simulink model "35-Bus_Network_Electricity_Transmission_Model"  (R2023b)
settings: Solver=VariableStepAuto  StartTime=0.0  StopTime=10  RelTol=1e-3
undefined symbols (not defined in the file): D1, D11, Delta
libraries: spsSeriesRLCBranchLib x47, spsLoadFlowBusLib x35, spsThreePhaseSeriesRLCLoadLib x27, spsDistributedParametersLineLib x22, spsGenericPowerSystemStabilizerLib x20, spsThreePhaseTransformerTwoWindingsLib x19, spsThreePhaseVIMeasurementLib x13, spsSynchronousMachinepuStandardLib x10, spsExcitationSystemLib x10, spsHydraulicTurbineandGovernorLib x10, spsThreePhaseParallelRLCLoadLib x4, spsGroundLib x3
(part 2 of 7)

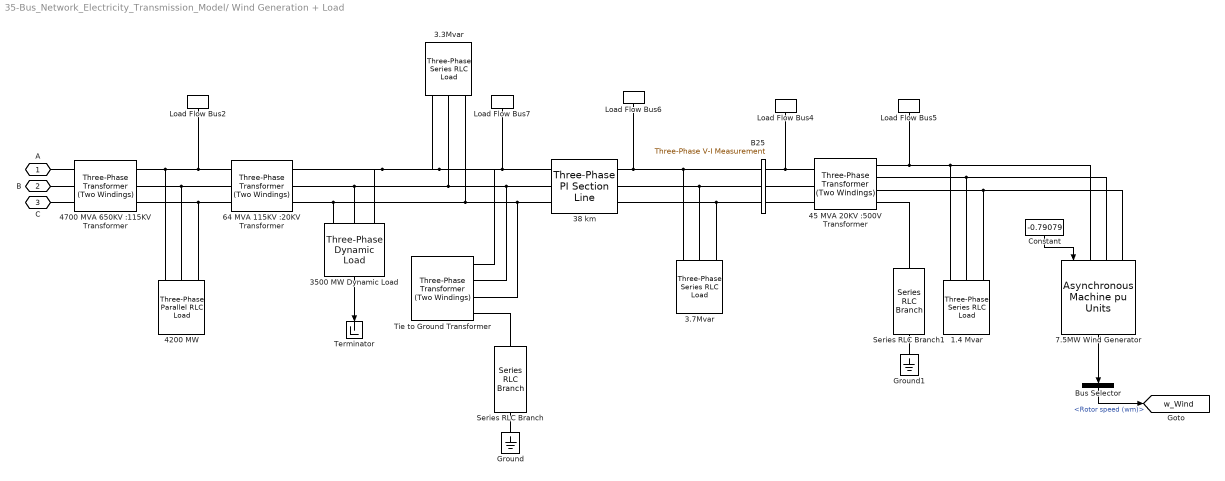
== system 35-Bus_Network_Electricity_Transmission_Model/ Wind Generation + Load ==
  " 64 MVA 115KV :20KV Transformer " : spsThreePhaseTransformerTwoWindingsLib/Three-Phase Transformer (Two Windings)  Winding1Connection=Yg  Winding2Connection=Delta (D1)  CoreType=Three single-phase transformers  SetSaturation=off  Hysteresis=off  DataFile='hysteresis'  SetInitialFlux=off  Measurements=None  UNITS=pu  NominalPower=[ 64e6 , 60 ]  Winding1=[ 115e3 , 0.002 , 0.08 ]  Winding2=[ 20e3 , 0.002 , 0.08 ]  Rm=500  Lm=500  L0=0.5  Saturation=[ 0,0 ; 0.0024,1.2 ; 1.0,1.52 ]  InitialFluxes=[ 0.8 , -0.8 , 0.7 ]  BreakLoop=off  DiscreteSolver=Trapezoidal iterative  DataType=off  TransfoNumber=1
  " Tie to Ground Transformer " : spsThreePhaseTransformerTwoWindingsLib/Three-Phase Transformer (Two Windings)  Winding1Connection=Yn  Winding2Connection=Delta (D11)  CoreType=Three single-phase transformers  SetSaturation=off  Hysteresis=off  DataFile='hysteresis'  SetInitialFlux=off  Measurements=None  UNITS=pu  NominalPower=[ 5600e6 , 60 ]  Winding1=[ 13.8e3 , 0.002 , 0.08 ]  Winding2=[ 735e3 , 0.002 , 0.08 ]  Rm=500  Lm=500  L0=0.5  Saturation=[ 0,0 ; 0.0024,1.2 ; 1.0,1.52 ]  InitialFluxes=[ 0.8 , -0.8 , 0.7 ]  BreakLoop=off  DiscreteSolver=Trapezoidal iterative  DataType=off  TransfoNumber=1
  1.4 Mvar : spsThreePhaseSeriesRLCLoadLib/Three-Phase Series RLC Load  LConnTagsString=A|B|C  Configuration=Y (grounded)  NominalVoltage=1000  Vabc=[1e3 1e3 1e3]  Vabcp=[1e3 1e3 1e3]  NominalFrequency=60  UnbalancedPower=off  ActivePower=0  InductivePower=0  CapacitivePower=1.4e6  Pabc=[10e3 9e3 11e3]  QLabc=[100 90 110]  QCabc=[100 90 110]  Pabcp=[10e3 9e3 11e3]  QLabcp=[100 90 110]  QCabcp=[100 90 110]  Measurements=None  LoadType=constant Z
  3.3Mvar : spsThreePhaseSeriesRLCLoadLib/Three-Phase Series RLC Load  LConnTagsString=A|B|C  Configuration=Y (grounded)  NominalVoltage=1000  Vabc=[1e3 1e3 1e3]  Vabcp=[1e3 1e3 1e3]  NominalFrequency=60  UnbalancedPower=off  ActivePower=0  InductivePower=0  CapacitivePower=3.3e6  Pabc=[10e3 9e3 11e3]  QLabc=[100 90 110]  QCabc=[100 90 110]  Pabcp=[10e3 9e3 11e3]  QLabcp=[100 90 110]  QCabcp=[100 90 110]  Measurements=None  LoadType=constant Z
  3.7Mvar : spsThreePhaseSeriesRLCLoadLib/Three-Phase Series RLC Load  LConnTagsString=A|B|C  Configuration=Y (grounded)  NominalVoltage=1000  Vabc=[1e3 1e3 1e3]  Vabcp=[1e3 1e3 1e3]  NominalFrequency=60  UnbalancedPower=off  ActivePower=0  InductivePower=0  CapacitivePower=3.7e6  Pabc=[10e3 9e3 11e3]  QLabc=[100 90 110]  QCabc=[100 90 110]  Pabcp=[10e3 9e3 11e3]  QLabcp=[100 90 110]  QCabcp=[100 90 110]  Measurements=None  LoadType=constant Z
  3500 MW Dynamic Load : spsThreePhaseDynamicLoadLib/Three-Phase Dynamic Load  NominalVoltage=[ 500e3 60 ]  ActiveReactivePowers=[3500e6 0]  PositiveSequence=[0.994 -11.8]  ExternalControl=off  NpNq=[1.3 2]  TimeConstants="[0  0  0  0]"  MinimumVoltage=0.7  Tfilter=1e-4  LoadFlowParameters=[4,0,0,0,0]
      settings: LibrarySourceBlock=|
      | sps_lib/Passives/Three-Phase
      | Dynamic Load
  38 km : spsThreePhasePISectionLineLib/Three-Phase PI Section Line  LConnTagsString=a|b|c  RConnTagsString=A|B|C  Length=38  Frequency=60  Resistances=[ 0.01273 0.3864]/6  Inductances="[ 0.9337e-3  4.1264e-3]/6"  Capacitances=[12.74e-9 7.751e-9]*6
  4200 MW : spsThreePhaseParallelRLCLoadLib/Three-Phase Parallel RLC Load  LConnTagsString=A|B|C  Configuration=Y (grounded)  NominalVoltage=1000  Vabc=[1e3 1e3 1e3]  Vabcp=[1e3 1e3 1e3]  NominalFrequency=60  UnbalancedPower=off  ActivePower=4200e6  InductivePower=0  CapacitivePower=0  Pabc=[10e3 9e3 11e3]  QLabc=[100 90 110]  QCabc=[100 90 110]  Pabcp=[10e3 9e3 11e3]  QLabcp=[100 90 110]  QCabcp=[100 90 110]  Measurements=None  LoadType=constant Z
  "45 MVA 20KV :500V Transformer " : spsThreePhaseTransformerTwoWindingsLib/Three-Phase Transformer (Two Windings)  Winding1Connection=Yg  Winding2Connection=Yn  CoreType=Three single-phase transformers  SetSaturation=off  Hysteresis=off  DataFile='hysteresis'  SetInitialFlux=off  Measurements=None  UNITS=pu  NominalPower=[ 12e6 , 60 ]  Winding1=[ 20e3 , 0.002 , 0.08 ]  Winding2=[ 500 , 0.002 , 0.08 ]  Rm=500  Lm=500  L0=0.5  Saturation=[ 0,0 ; 0.0024,1.2 ; 1.0,1.52 ]  InitialFluxes=[ 0.8 , -0.8 , 0.7 ]  BreakLoop=off  DiscreteSolver=Trapezoidal iterative  DataType=off  TransfoNumber=1
  "4700 MVA 650KV :115KV Transformer " : spsThreePhaseTransformerTwoWindingsLib/Three-Phase Transformer (Two Windings)  Winding1Connection=Yg  Winding2Connection=Delta (D1)  CoreType=Three single-phase transformers  SetSaturation=off  Hysteresis=off  DataFile='hysteresis'  SetInitialFlux=off  Measurements=None  UNITS=pu  NominalPower=[ 4700e6 , 60 ]  Winding1=[ 650e3 , 0.002 , 0.08 ]  Winding2=[ 115e3 , 0.002 , 0.08 ]  Rm=500  Lm=500  L0=0.5  Saturation=[ 0,0 ; 0.0024,1.2 ; 1.0,1.52 ]  InitialFluxes=[ 0.8 , -0.8 , 0.7 ]  BreakLoop=off  DiscreteSolver=Trapezoidal iterative  DataType=off  TransfoNumber=1
  7.5MW Wind Generator : spsAsynchronousMachinepuUnitsLib/Asynchronous Machine pu Units  RotorType=Squirrel-cage  PresetModel=No  MechanicalLoad=Torque Tm  ShowDetailedParameters=on  ReferenceFrame=Rotor  Units=pu  MeasurementBus=off  NominalParameters=[8500 500 60]  VoltageRatio=1  Stator=[0.01965 0.0397]  Rotor=[0.01909 0.0397]  Cage1=[0.01909 0.0397]  Cage2=[0.01909 0.0397]  Lm=6.354  Mechanical=[0.09526 0.05479 2]  PolePairs=2  InitialConditions=[ -0.004758 0 0.749638 0.749638 0.749638 128.64 8.64 248.64 ]  SimulateSaturation=off  Saturation="[0.212,0.4201,0.8125,1.0979,1.4799,2.2457,3.2586,4.5763,6.4763 ;   0.5,0.7,0.9,1,1.1,1.2 ,1.3,1.4,1.5]"  LoadFlowParameters=0  TsPowergui=0  TsBlock=-1  IterativeModel=Trapezoidal non iterative  IterativeDiscreteModel=Trapezoidal non iterative  Pmec=75e5
      settings: LibrarySourceBlock=|
      | sps_lib/Electrical Machines/Asynchronous Machine
      | pu Units
  B25 : spsThreePhaseVIMeasurementLib/Three-Phase V-I Measurement  VoltageMeasurement=no  SetLabelV=off  LabelV=Vabc  Vpu=off  VpuLL=off  CurrentMeasurement=no  SetLabelI=off  LabelI=Iabc  Ipu=off  Pbase=100e6  Vbase=500e3  OutputType=Complex  PhasorSimulation=off  PSBequivalent=0
  Bus Selector : BusSelector  OutputSignals=Mechanical.Rotor speed (wm)
  Constant : Constant  Value=-0.79079
  Ground : spsGroundLib/Ground  LConnTagsString=a
  Ground1 : spsGroundLib/Ground  LConnTagsString=a
  Load Flow Bus2 : spsLoadFlowBusLib/Load Flow Bus  LConnTagsString=a  Phases=single  Connectors=on one side  ID=BUS_28  Vbase=650e3  Vref=1  Vangle=0  VLF=1  VLFb=1  VLFc=1  angleLF=0  angleLFb=0  angleLFc=0
  Load Flow Bus4 : spsLoadFlowBusLib/Load Flow Bus  LConnTagsString=a  Phases=single  Connectors=on one side  ID=BUS_31  Vbase=20e3  Vref=1  Vangle=0  VLF=1  VLFb=1  VLFc=1  angleLF=0  angleLFb=0  angleLFc=0
  Load Flow Bus5 : spsLoadFlowBusLib/Load Flow Bus  LConnTagsString=a  Phases=single  Connectors=on one side  ID=BUS_32  Vbase=450  Vref=1  Vangle=0  VLF=1  VLFb=1  VLFc=1  angleLF=0  angleLFb=0  angleLFc=0
  Load Flow Bus6 : spsLoadFlowBusLib/Load Flow Bus  LConnTagsString=a  Phases=single  Connectors=on one side  ID=BUS_30  Vbase=20e3  Vref=1  Vangle=0  VLF=1  VLFb=1  VLFc=1  angleLF=0  angleLFb=0  angleLFc=0
  Load Flow Bus7 : spsLoadFlowBusLib/Load Flow Bus  LConnTagsString=a  Phases=single  Connectors=on one side  ID=BUS_29  Vbase=20e3  Vref=1  Vangle=0  VLF=1  VLFb=1  VLFc=1  angleLF=0  angleLFb=0  angleLFc=0
  Series RLC Branch : spsSeriesRLCBranchLib/Series RLC Branch  LConnTagsString=__new0  RConnTagsString=__new0  BranchType=R  Resistance=4.1  Inductance=0  SetiL0=off  InitialCurrent=0  Capacitance=0  Setx0=off  InitialVoltage=0  Measurements=None
  Series RLC Branch1 : spsSeriesRLCBranchLib/Series RLC Branch  LConnTagsString=__new0  RConnTagsString=__new0  BranchType=R  Resistance=19.4  Inductance=0  SetiL0=off  InitialCurrent=0  Capacitance=0  Setx0=off  InitialVoltage=0  Measurements=None
  Terminator : Terminator
  A : PMIOPort  Side=Left
  B : PMIOPort  Port=2  Side=Left
  C : PMIOPort  Port=3  Side=Left
  tag scope: w_Wind=global
  wires:
  3500 MW Dynamic Load/1 -> Terminator/1
  Constant/1 -> 7.5MW Wind Generator/1
  Bus Selector/1 -> [w_Wind]  "<Rotor speed (wm)>"
  7.5MW Wind Generator/1 -> Bus Selector/1
  connections:
  Load Flow Bus6/LConn1 -- 3.7Mvar/LConn1 -- B25/RConn1 -- 38 km/RConn1
  " Tie to Ground Transformer "/LConn4 -- Series RLC Branch/LConn1
  3.7Mvar/LConn2 -- 38 km/RConn2 -- B25/RConn2
  "4700 MVA 650KV :115KV Transformer "/RConn1 -- " 64 MVA 115KV :20KV Transformer "/LConn1 -- Load Flow Bus2/LConn1 -- 4200 MW/LConn1
  "4700 MVA 650KV :115KV Transformer "/RConn2 -- " 64 MVA 115KV :20KV Transformer "/LConn2 -- 4200 MW/LConn2
  3.7Mvar/LConn3 -- 38 km/RConn3 -- B25/RConn3
  7.5MW Wind Generator/LConn3 -- "45 MVA 20KV :500V Transformer "/RConn3 -- 1.4 Mvar/LConn3
  "4700 MVA 650KV :115KV Transformer "/RConn3 -- " 64 MVA 115KV :20KV Transformer "/LConn3 -- 4200 MW/LConn3
  38 km/LConn2 -- " Tie to Ground Transformer "/LConn2 -- 3500 MW Dynamic Load/LConn2 -- " 64 MVA 115KV :20KV Transformer "/RConn2 -- 3.3Mvar/LConn2
  B25/LConn2 -- "45 MVA 20KV :500V Transformer "/LConn2
  "45 MVA 20KV :500V Transformer "/LConn1 -- Load Flow Bus4/LConn1 -- B25/LConn1
  7.5MW Wind Generator/LConn2 -- "45 MVA 20KV :500V Transformer "/RConn2 -- 1.4 Mvar/LConn2
  "45 MVA 20KV :500V Transformer "/RConn1 -- Load Flow Bus5/LConn1 -- 1.4 Mvar/LConn1 -- 7.5MW Wind Generator/LConn1
  38 km/LConn3 -- " Tie to Ground Transformer "/LConn3 -- 3500 MW Dynamic Load/LConn3 -- " 64 MVA 115KV :20KV Transformer "/RConn3 -- 3.3Mvar/LConn3
  38 km/LConn1 -- " Tie to Ground Transformer "/LConn1 -- 3500 MW Dynamic Load/LConn1 -- " 64 MVA 115KV :20KV Transformer "/RConn1 -- 3.3Mvar/LConn1 -- Load Flow Bus7/LConn1
  Series RLC Branch1/RConn1 -- Ground1/LConn1
  B25/LConn3 -- "45 MVA 20KV :500V Transformer "/LConn3
  Series RLC Branch1/LConn1 -- "45 MVA 20KV :500V Transformer "/RConn4
  Series RLC Branch/RConn1 -- Ground/LConn1
  "4700 MVA 650KV :115KV Transformer "/LConn1 -- A/RConn1
  "4700 MVA 650KV :115KV Transformer "/LConn3 -- C/RConn1
  "4700 MVA 650KV :115KV Transformer "/LConn2 -- B/RConn1

== system 35-Bus_Network_Electricity_Transmission_Model/Cs MPOD ==
  Series RLC Branch : spsSeriesRLCBranchLib/Series RLC Branch  LConnTagsString=__new0  RConnTagsString=__new0  BranchType=C  Resistance=1  Inductance=1e-3  SetiL0=off  InitialCurrent=0  Capacitance=0.00049736  Setx0=off  InitialVoltage=0  Measurements=None
  Series RLC Branch1 : spsSeriesRLCBranchLib/Series RLC Branch  LConnTagsString=__new0  RConnTagsString=__new0  BranchType=C  Resistance=1  Inductance=1e-3  SetiL0=off  InitialCurrent=0  Capacitance=0.00049736  Setx0=off  InitialVoltage=0  Measurements=None
  Series RLC Branch2 : spsSeriesRLCBranchLib/Series RLC Branch  LConnTagsString=__new0  RConnTagsString=__new0  BranchType=C  Resistance=1  Inductance=1e-3  SetiL0=off  InitialCurrent=0  Capacitance=0.00049736  Setx0=off  InitialVoltage=0  Measurements=None
  A : PMIOPort  Side=Left
  A1 : PMIOPort  Port=2  Side=Right
  B : PMIOPort  Port=3  Side=Left
  B1 : PMIOPort  Port=4  Side=Right
  C : PMIOPort  Port=5  Side=Left
  C1 : PMIOPort  Port=6  Side=Right
  connections:
  A1/RConn1 -- Series RLC Branch/RConn1
  B1/RConn1 -- Series RLC Branch1/RConn1
  A/RConn1 -- Series RLC Branch/LConn1
  C/RConn1 -- Series RLC Branch2/LConn1
  B/RConn1 -- Series RLC Branch1/LConn1
  C1/RConn1 -- Series RLC Branch2/RConn1

== system 35-Bus_Network_Electricity_Transmission_Model/Cs OSIS ==
  Series RLC Branch : spsSeriesRLCBranchLib/Series RLC Branch  LConnTagsString=__new0  RConnTagsString=__new0  BranchType=C  Resistance=1  Inductance=1e-3  SetiL0=off  InitialCurrent=0  Capacitance=0.00049736  Setx0=off  InitialVoltage=0  Measurements=None
  Series RLC Branch1 : spsSeriesRLCBranchLib/Series RLC Branch  LConnTagsString=__new0  RConnTagsString=__new0  BranchType=C  Resistance=1  Inductance=1e-3  SetiL0=off  InitialCurrent=0  Capacitance=0.00049736  Setx0=off  InitialVoltage=0  Measurements=None
  Series RLC Branch2 : spsSeriesRLCBranchLib/Series RLC Branch  LConnTagsString=__new0  RConnTagsString=__new0  BranchType=C  Resistance=1  Inductance=1e-3  SetiL0=off  InitialCurrent=0  Capacitance=0.00049736  Setx0=off  InitialVoltage=0  Measurements=None
  A : PMIOPort  Side=Left
  A1 : PMIOPort  Port=2  Side=Right
  B : PMIOPort  Port=3  Side=Left
  B1 : PMIOPort  Port=4  Side=Right
  C : PMIOPort  Port=5  Side=Left
  C1 : PMIOPort  Port=6  Side=Right
  connections:
  A1/RConn1 -- Series RLC Branch/RConn1
  B1/RConn1 -- Series RLC Branch1/RConn1
  A/RConn1 -- Series RLC Branch/LConn1
  C/RConn1 -- Series RLC Branch2/LConn1
  B/RConn1 -- Series RLC Branch1/LConn1
  C1/RConn1 -- Series RLC Branch2/RConn1

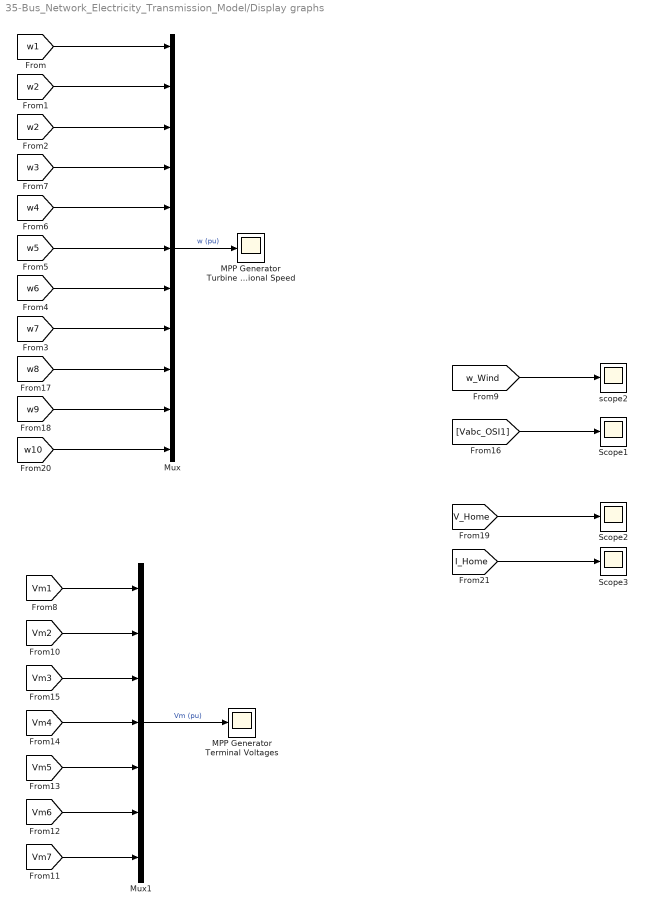
== system 35-Bus_Network_Electricity_Transmission_Model/Display graphs ==
  MPP Generator Terminal Voltages : Scope
  MPP Generator Turbine Rotational Speed : Scope
  Mux : Mux  Inputs=11
  Mux1 : Mux  Inputs=7
  Scope1 : Scope
  Scope2 : Scope
  Scope3 : Scope
  scope2 : Scope
  wires:
  [w2] -> Mux/2
  [Vm5] -> Mux1/5
  [Vm3] -> Mux1/3
  [Vm1] -> Mux1/1
  [Vm4] -> Mux1/4
  [Vm6] -> Mux1/6
  [Vm2] -> Mux1/2
  [w6] -> Mux/7
  [Vm7] -> Mux1/7
  Mux1/1 -> MPP Generator Terminal Voltages/1  "Vm (pu)"
  [w2] -> Mux/3
  [w1] -> Mux/1
  [w3] -> Mux/4
  [w4] -> Mux/5
  [w_Wind] -> scope2/1
  [Vabc_OSI1] -> Scope1/1
  Mux/1 -> MPP Generator Turbine Rotational Speed/1  "w (pu)"
  [w7] -> Mux/8
  [w5] -> Mux/6
  [w8] -> Mux/9
  [w9] -> Mux/10
  [w10] -> Mux/11
  [V_Home] -> Scope2/1
  [I_Home] -> Scope3/1

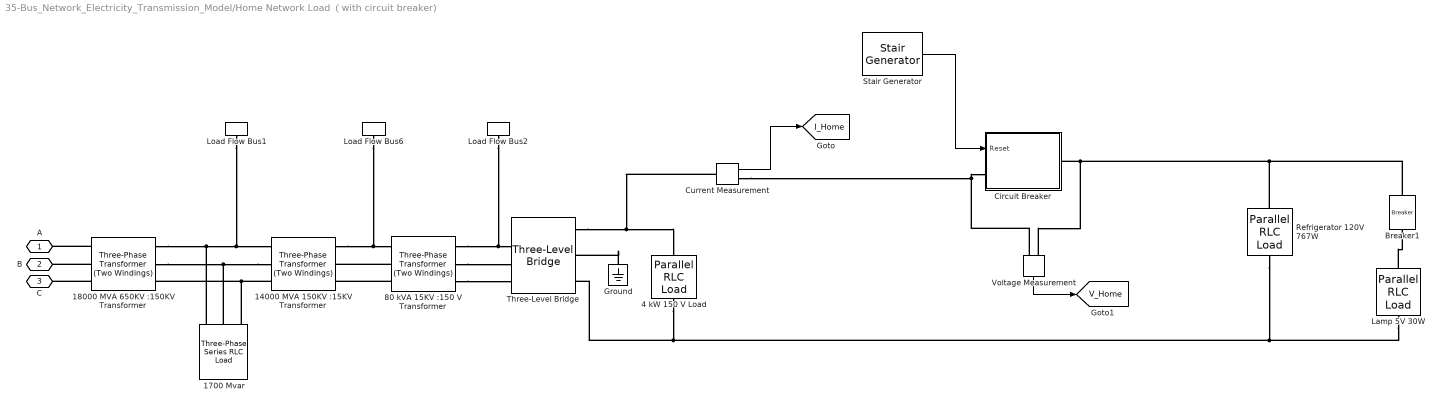
== system 35-Bus_Network_Electricity_Transmission_Model/Home Network Load （with circuit breaker) ==
  " Refrigerator 120V 767W" : spsParallelRLCLoadLib/Parallel RLC Load  LConnTagsString=a  RConnTagsString=__new0  NominalVoltage=1000  NominalFrequency=60  ActivePower=10e3  InductivePower=100  CapacitivePower=100  Setx0=off  InitialVoltage=0  SetiL0=off  InitialCurrent=0  Measurements=None  LoadType=constant Z
      settings: AttributesFormatString=\n  LibrarySourceBlock=sps_lib/Passives/Parallel RLC Load
  "14000 MVA 150KV :15KV Transformer " : spsThreePhaseTransformerTwoWindingsLib/Three-Phase Transformer (Two Windings)  Winding1Connection=Yg  Winding2Connection=Delta (D1)  CoreType=Three single-phase transformers  SetSaturation=off  Hysteresis=off  DataFile='hysteresis'  SetInitialFlux=off  Measurements=None  UNITS=pu  NominalPower=[ 14000e6 , 60 ]  Winding1=[ 150e3 , 0.002 , 0.08 ]  Winding2=[ 15e3 , 0.002 , 0.08 ]  Rm=500  Lm=500  L0=0.5  Saturation=[ 0,0 ; 0.0024,1.2 ; 1.0,1.52 ]  InitialFluxes=[ 0.8 , -0.8 , 0.7 ]  BreakLoop=off  DiscreteSolver=Trapezoidal iterative  DataType=off  TransfoNumber=1
  1700 Mvar : spsThreePhaseSeriesRLCLoadLib/Three-Phase Series RLC Load  LConnTagsString=A|B|C  Configuration=Y (grounded)  NominalVoltage=1000  Vabc=[1e3 1e3 1e3]  Vabcp=[1e3 1e3 1e3]  NominalFrequency=60  UnbalancedPower=off  ActivePower=0  InductivePower=0  CapacitivePower=1700e6  Pabc=[10e3 9e3 11e3]  QLabc=[100 90 110]  QCabc=[100 90 110]  Pabcp=[10e3 9e3 11e3]  QLabcp=[100 90 110]  QCabcp=[100 90 110]  Measurements=None  LoadType=constant Z
  "18000 MVA 650KV :150KV Transformer " : spsThreePhaseTransformerTwoWindingsLib/Three-Phase Transformer (Two Windings)  Winding1Connection=Yg  Winding2Connection=Delta (D1)  CoreType=Three single-phase transformers  SetSaturation=off  Hysteresis=off  DataFile='hysteresis'  SetInitialFlux=off  Measurements=None  UNITS=pu  NominalPower=[ 18000e6 , 60 ]  Winding1=[ 650e3 , 0.002 , 0.08 ]  Winding2=[ 150e3 , 0.002 , 0.08 ]  Rm=500  Lm=500  L0=0.5  Saturation=[ 0,0 ; 0.0024,1.2 ; 1.0,1.52 ]  InitialFluxes=[ 0.8 , -0.8 , 0.7 ]  BreakLoop=off  DiscreteSolver=Trapezoidal iterative  DataType=off  TransfoNumber=1
  4 kW 150 V Load : spsParallelRLCLoadLib/Parallel RLC Load  LConnTagsString=a  RConnTagsString=__new0  NominalVoltage=150  NominalFrequency=60  ActivePower=4e3  InductivePower=100  CapacitivePower=100  Setx0=off  InitialVoltage=0  SetiL0=off  InitialCurrent=0  Measurements=None  LoadType=constant Z
      settings: AttributesFormatString=\n  LibrarySourceBlock=sps_lib/Passives/Parallel RLC Load
  "80 kVA 15KV :150 V Transformer " : spsThreePhaseTransformerTwoWindingsLib/Three-Phase Transformer (Two Windings)  Winding1Connection=Yg  Winding2Connection=Yg  CoreType=Three single-phase transformers  SetSaturation=off  Hysteresis=off  DataFile='hysteresis'  SetInitialFlux=off  Measurements=None  UNITS=pu  NominalPower=[ 80e3 , 60 ]  Winding1=[ 15e3 , 0.002 , 0.08 ]  Winding2=[ 150 , 0.002 , 0.08 ]  Rm=500  Lm=500  L0=0.5  Saturation=[ 0,0 ; 0.0024,1.2 ; 1.0,1.52 ]  InitialFluxes=[ 0.8 , -0.8 , 0.7 ]  BreakLoop=off  DiscreteSolver=Trapezoidal iterative  DataType=off  TransfoNumber=1
  Breaker1 : spsBreakerLib/Breaker  InitialState=0  SwitchingTimes=[.05 0.1]  External=off  BreakerResistance=1e-5  SnubberResistance=1e6  SnubberCapacitance=inf  Measurements=None  MoreParameters=off  NoBreakLoop=off
      settings: AttributesFormatString=\n
  Circuit Breaker : Subsystem
  Current Measurement : spsCurrentMeasurementLib/Current Measurement  PhasorSimulation=off  OutputType=Complex  PSBequivalent=0
  Ground : spsGroundLib/Ground  LConnTagsString=a
  Lamp 5V 30W : spsParallelRLCLoadLib/Parallel RLC Load  LConnTagsString=a  RConnTagsString=__new0  NominalVoltage=1000  NominalFrequency=60  ActivePower=10e3  InductivePower=100  CapacitivePower=100  Setx0=off  InitialVoltage=0  SetiL0=off  InitialCurrent=0  Measurements=None  LoadType=constant Z
      settings: AttributesFormatString=\n  LibrarySourceBlock=sps_lib/Passives/Parallel RLC Load
  Load Flow Bus1 : spsLoadFlowBusLib/Load Flow Bus  LConnTagsString=a  Phases=single  Connectors=on one side  ID=BUS_33  Vbase=150e3  Vref=1  Vangle=0  VLF=1  VLFb=1  VLFc=1  angleLF=0  angleLFb=0  angleLFc=0
  Load Flow Bus2 : spsLoadFlowBusLib/Load Flow Bus  LConnTagsString=a  Phases=single  Connectors=on one side  ID=BUS_35  Vbase=150  Vref=1  Vangle=0  VLF=1  VLFb=1  VLFc=1  angleLF=0  angleLFb=0  angleLFc=0
  Load Flow Bus6 : spsLoadFlowBusLib/Load Flow Bus  LConnTagsString=a  Phases=single  Connectors=on one side  ID=BUS_34  Vbase=15e3  Vref=1  Vangle=0  VLF=1  VLFb=1  VLFc=1  angleLF=0  angleLFb=0  angleLFc=0
  Stair Generator : eeStairGenerator/Stair Generator  LabelModeActiveChoice=Continuous  TimeInput=[0 3e-3 15e-3]  AmplitudeInput=[1 0 1]  SampleTime=0  RepeatPattern=off  OutDataTypeStr=double
      settings: LibrarySourceBlock=ee_sl_lib/General Control/Stair Generator
  Three-Level Bridge : spsThreeLevelBridgeLib/Three-Level Bridge  Arms=3  SnubberResistance=1e5  SbubberCapacitance=inf  Device=GTO / Diodes  Ron=1e-3  ForwardVoltages="[  0  0  ]"  Measurements=None
      settings: LibrarySourceBlock=sps_lib/Power Electronics/Three-Level Bridge
  Voltage Measurement : spsVoltageMeasurementLib/Voltage Measurement  PhasorSimulation=off  OutputType=Complex  PSBequivalent=0
  A : PMIOPort  Side=Left
  B : PMIOPort  Port=2  Side=Left
  C : PMIOPort  Port=3  Side=Left
  tag scope: I_Home=global, V_Home=global
  wires:
  Stair Generator/1 -> Circuit Breaker/1("Reset ")
  Current Measurement/1 -> [I_Home]
  Voltage Measurement/1 -> [V_Home]
  connections:
  "18000 MVA 650KV :150KV Transformer "/RConn1 -- 1700 Mvar/LConn1 -- "14000 MVA 150KV :15KV Transformer "/LConn1 -- Load Flow Bus1/LConn1
  "18000 MVA 650KV :150KV Transformer "/LConn1 -- A/RConn1
  "18000 MVA 650KV :150KV Transformer "/RConn3 -- "14000 MVA 150KV :15KV Transformer "/LConn3 -- 1700 Mvar/LConn3
  "14000 MVA 150KV :15KV Transformer "/LConn2 -- "18000 MVA 650KV :150KV Transformer "/RConn2 -- 1700 Mvar/LConn2
  "18000 MVA 650KV :150KV Transformer "/LConn2 -- B/RConn1
  "18000 MVA 650KV :150KV Transformer "/LConn3 -- C/RConn1
  "14000 MVA 150KV :15KV Transformer "/RConn1 -- Load Flow Bus6/LConn1 -- "80 kVA 15KV :150 V Transformer "/LConn1
  "80 kVA 15KV :150 V Transformer "/LConn2 -- "14000 MVA 150KV :15KV Transformer "/RConn2
  "80 kVA 15KV :150 V Transformer "/LConn3 -- "14000 MVA 150KV :15KV Transformer "/RConn3
  "80 kVA 15KV :150 V Transformer "/RConn1 -- Load Flow Bus2/LConn1 -- Three-Level Bridge/LConn1
  "80 kVA 15KV :150 V Transformer "/RConn2 -- Three-Level Bridge/LConn2
  "80 kVA 15KV :150 V Transformer "/RConn3 -- Three-Level Bridge/LConn3
  Three-Level Bridge/RConn1 -- Current Measurement/LConn1 -- 4 kW 150 V Load/LConn1
  4 kW 150 V Load/RConn1 -- Lamp 5V 30W/RConn1 -- " Refrigerator 120V 767W"/RConn1 -- Three-Level Bridge/RConn3
  Voltage Measurement/LConn2 -- Breaker1/LConn1 -- " Refrigerator 120V 767W"/LConn1 -- Circuit Breaker/RConn1
  Ground/LConn1 -- Three-Level Bridge/RConn2
  Voltage Measurement/LConn1 -- Circuit Breaker/LConn1 -- Current Measurement/RConn1
  Lamp 5V 30W/LConn1 -- Breaker1/RConn1

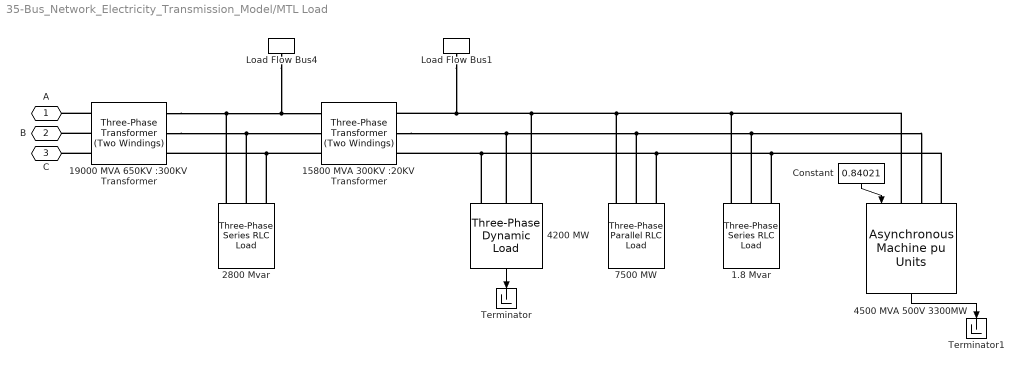
== system 35-Bus_Network_Electricity_Transmission_Model/MTL Load ==
  1.8 Mvar : spsThreePhaseSeriesRLCLoadLib/Three-Phase Series RLC Load  LConnTagsString=A|B|C  Configuration=Y (grounded)  NominalVoltage=1000  Vabc=[1e3 1e3 1e3]  Vabcp=[1e3 1e3 1e3]  NominalFrequency=60  UnbalancedPower=off  ActivePower=0  InductivePower=0  CapacitivePower=1.8e6  Pabc=[10e3 9e3 11e3]  QLabc=[100 90 110]  QCabc=[100 90 110]  Pabcp=[10e3 9e3 11e3]  QLabcp=[100 90 110]  QCabcp=[100 90 110]  Measurements=None  LoadType=constant Z
  "15800 MVA 300KV :20KV Transformer " : spsThreePhaseTransformerTwoWindingsLib/Three-Phase Transformer (Two Windings)  Winding1Connection=Yg  Winding2Connection=Delta (D1)  CoreType=Three single-phase transformers  SetSaturation=off  Hysteresis=off  DataFile='hysteresis'  SetInitialFlux=off  Measurements=None  UNITS=pu  NominalPower=[ 15800e6 , 60 ]  Winding1=[ 300e3 , 0.002 , 0.08 ]  Winding2=[ 20e3 , 0.002 , 0.08 ]  Rm=500  Lm=500  L0=0.5  Saturation=[ 0,0 ; 0.0024,1.2 ; 1.0,1.52 ]  InitialFluxes=[ 0.8 , -0.8 , 0.7 ]  BreakLoop=off  DiscreteSolver=Trapezoidal iterative  DataType=off  TransfoNumber=1
  "19000 MVA 650KV :300KV Transformer " : spsThreePhaseTransformerTwoWindingsLib/Three-Phase Transformer (Two Windings)  Winding1Connection=Yg  Winding2Connection=Delta (D1)  CoreType=Three single-phase transformers  SetSaturation=off  Hysteresis=off  DataFile='hysteresis'  SetInitialFlux=off  Measurements=None  UNITS=pu  NominalPower=[ 19000e6 , 60 ]  Winding1=[ 650e3 , 0.002 , 0.08 ]  Winding2=[ 300e3 , 0.002 , 0.08 ]  Rm=500  Lm=500  L0=0.5  Saturation=[ 0,0 ; 0.0024,1.2 ; 1.0,1.52 ]  InitialFluxes=[ 0.8 , -0.8 , 0.7 ]  BreakLoop=off  DiscreteSolver=Trapezoidal iterative  DataType=off  TransfoNumber=1
  2800 Mvar : spsThreePhaseSeriesRLCLoadLib/Three-Phase Series RLC Load  LConnTagsString=A|B|C  Configuration=Y (grounded)  NominalVoltage=1000  Vabc=[1e3 1e3 1e3]  Vabcp=[1e3 1e3 1e3]  NominalFrequency=60  UnbalancedPower=off  ActivePower=0  InductivePower=0  CapacitivePower=2800e6  Pabc=[10e3 9e3 11e3]  QLabc=[100 90 110]  QCabc=[100 90 110]  Pabcp=[10e3 9e3 11e3]  QLabcp=[100 90 110]  QCabcp=[100 90 110]  Measurements=None  LoadType=constant Z
  4200 MW : spsThreePhaseDynamicLoadLib/Three-Phase Dynamic Load  NominalVoltage=[ 500e3 60 ]  ActiveReactivePowers=[4200e6 0]  PositiveSequence=[0.994 -11.8]  ExternalControl=off  NpNq=[1.3 2]  TimeConstants="[0  0  0  0]"  MinimumVoltage=0.7  Tfilter=1e-4  LoadFlowParameters=[4,0,0,0,0]
      settings: LibrarySourceBlock=|
      | sps_lib/Passives/Three-Phase
      | Dynamic Load
  4500 MVA 500V 3300MW : spsAsynchronousMachinepuUnitsLib/Asynchronous Machine pu Units  RotorType=Squirrel-cage  PresetModel=No  MechanicalLoad=Torque Tm  ShowDetailedParameters=on  ReferenceFrame=Rotor  Units=pu  MeasurementBus=off  NominalParameters=[4500 500 60]  VoltageRatio=1  Stator=[0.01965 0.0397]  Rotor=[0.01909 0.0397]  Cage1=[0.01909 0.0397]  Cage2=[0.01909 0.0397]  Lm=2.57  Mechanical=[0.09526 0.05479 2]  PolePairs=2  InitialConditions=[ -0.004758 0 0.749638 0.749638 0.749638 128.64 8.64 248.64 ]  SimulateSaturation=off  Saturation="[0.212,0.4201,0.8125,1.0979,1.4799,2.2457,3.2586,4.5763,6.4763 ;   0.5,0.7,0.9,1,1.1,1.2 ,1.3,1.4,1.5]"  LoadFlowParameters=0  TsPowergui=0  TsBlock=-1  IterativeModel=Trapezoidal non iterative  IterativeDiscreteModel=Trapezoidal non iterative  Pmec=3300e6
      settings: LibrarySourceBlock=|
      | sps_lib/Electrical Machines/Asynchronous Machine
      | pu Units
  7500 MW : spsThreePhaseParallelRLCLoadLib/Three-Phase Parallel RLC Load  LConnTagsString=A|B|C  Configuration=Y (grounded)  NominalVoltage=1000  Vabc=[1e3 1e3 1e3]  Vabcp=[1e3 1e3 1e3]  NominalFrequency=60  UnbalancedPower=off  ActivePower=7500e6  InductivePower=0  CapacitivePower=0  Pabc=[10e3 9e3 11e3]  QLabc=[100 90 110]  QCabc=[100 90 110]  Pabcp=[10e3 9e3 11e3]  QLabcp=[100 90 110]  QCabcp=[100 90 110]  Measurements=None  LoadType=constant Z
  Constant : Constant  Value=0.84021
  Load Flow Bus1 : spsLoadFlowBusLib/Load Flow Bus  LConnTagsString=a  Phases=single  Connectors=on one side  ID=BUS_27  Vbase=20e3  Vref=1  Vangle=0  VLF=1  VLFb=1  VLFc=1  angleLF=0  angleLFb=0  angleLFc=0
  Load Flow Bus4 : spsLoadFlowBusLib/Load Flow Bus  LConnTagsString=a  Phases=single  Connectors=on one side  ID=BUS_26  Vbase=300e3  Vref=1  Vangle=0  VLF=1  VLFb=1  VLFc=1  angleLF=0  angleLFb=0  angleLFc=0
  Terminator : Terminator
  Terminator1 : Terminator
  A : PMIOPort  Side=Left
  B : PMIOPort  Port=2  Side=Left
  C : PMIOPort  Port=3  Side=Left
  wires:
  Constant/1 -> 4500 MVA 500V 3300MW/1
  4500 MVA 500V 3300MW/1 -> Terminator1/1
  4200 MW/1 -> Terminator/1
  connections:
  4500 MVA 500V 3300MW/LConn3 -- 1.8 Mvar/LConn3 -- 7500 MW/LConn3 -- 4200 MW/LConn3 -- "15800 MVA 300KV :20KV Transformer "/RConn3
  "19000 MVA 650KV :300KV Transformer "/RConn1 -- 2800 Mvar/LConn1 -- Load Flow Bus4/LConn1 -- "15800 MVA 300KV :20KV Transformer "/LConn1
  "15800 MVA 300KV :20KV Transformer "/LConn3 -- 2800 Mvar/LConn3 -- "19000 MVA 650KV :300KV Transformer "/RConn3
  4500 MVA 500V 3300MW/LConn1 -- 1.8 Mvar/LConn1 -- Load Flow Bus1/LConn1 -- "15800 MVA 300KV :20KV Transformer "/RConn1 -- 4200 MW/LConn1 -- 7500 MW/LConn1
  "15800 MVA 300KV :20KV Transformer "/RConn2 -- 7500 MW/LConn2 -- 4500 MVA 500V 3300MW/LConn2 -- 1.8 Mvar/LConn2 -- 4200 MW/LConn2
  "19000 MVA 650KV :300KV Transformer "/RConn2 -- 2800 Mvar/LConn2 -- "15800 MVA 300KV :20KV Transformer "/LConn2
  "19000 MVA 650KV :300KV Transformer "/LConn2 -- B/RConn1
  "19000 MVA 650KV :300KV Transformer "/LConn1 -- A/RConn1
  "19000 MVA 650KV :300KV Transformer "/LConn3 -- C/RConn1
